simulink model "Rate_Limit"  (Simulink 8.0)
settings: Solver=ode3  StartTime=0.0  StopTime=10.0  RelTol=1e-3
libraries: simulink x1
settings Model: Creator=Faradars  LastModifiedBy=Faradars

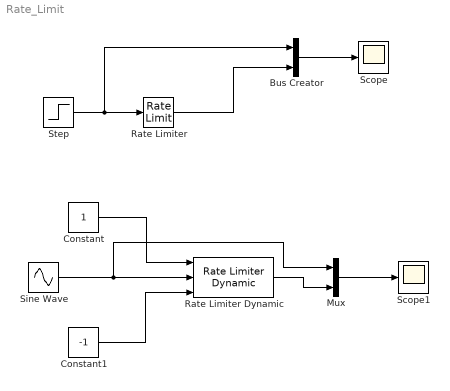
== system Rate_Limit ==
  Bus Creator : BusCreator  Inputs=2
  Constant : Constant
  Constant1 : Constant  Value=-1
  Mux : Mux  Inputs=2
  Rate Limiter : RateLimiter  RisingSlewLimit=0.5  FallingSlewLimit=-0.5  SampleTimeMode=inherited
  Rate Limiter Dynamic : simulink/Discontinuities/Rate Limiter Dynamic
  Scope : Scope
  Scope1 : Scope
  Sine Wave : Sin  Amplitude=2  Frequency=2  Phase=pi/2  SampleTime=0
  Step : Step  SampleTime=1
  wires:
  Sine Wave/1 -> Mux/1, Rate Limiter Dynamic/2
  Constant/1 -> Rate Limiter Dynamic/1
  Constant1/1 -> Rate Limiter Dynamic/3
  Mux/1 -> Scope1/1
  Rate Limiter Dynamic/1 -> Mux/2
  Bus Creator/1 -> Scope/1
  Rate Limiter/1 -> Bus Creator/2
  Step/1 -> Bus Creator/1, Rate Limiter/1
